simulink model "Just_The_Electrical_model"  (R2016a)
settings: Solver=VariableStepAuto  StartTime=0.0  StopTime=10.0  RelTol=1e-3
values from neighbouring files (symbols this model uses):
  BT = {}    [Electrical_model_settings.m]
  btc = {}    [Electrical_model_settings.m]
  col = {}    [Electrical_model_settings.m]
  elc = {}    [Electrical_model_settings.m]
  ess = {}    [Electrical_model_settings.m]
  fcc = {}    [Electrical_model_settings.m]
  flex = {}    [Electrical_model_settings.m]
  systemBase = {}    [Electrical_model_settings.m]
  wf = {}    [Electrical_model_settings.m]
  wt1 = {}    [Electrical_model_settings.m]
  wt2 = wt1    [Electrical_model_settings.m]
  wt3 = wt1    [Electrical_model_settings.m]
undefined symbols (not defined in the file or in its folder): avr, D1, Delta, DiscIntNeverNeededParam, f2ctrl, governor, interface, Lf1, sm, Ts, Ts_phy, Ts_sim, u0
libraries: powerlib x69, pwrsysBasic x68, simulink_extras x37, pwrsysVICtrl x22, powerlib_meascontrol x19, simulink x8, pwrsysVSrc x5, pwrsysTransf x5, pwrsys-matlab x1
(part 1 of 4)
settings Model: Creator=daniemot  LastModifiedBy=daniemot

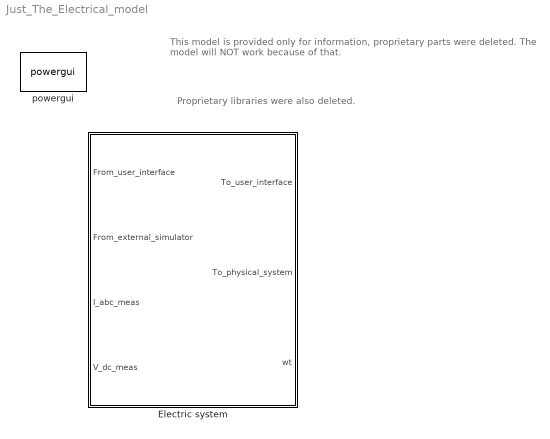
== system Just_The_Electrical_model ==
  note: Proprietary libraries were also deleted.
  note: This model is provided only for information, proprietary parts were deleted.
      | The model will NOT work because of that.
  Electric system : Subsystem
  powergui : powerlib/powergui  Priority=1  SimulationMode=Discrete  SolverType=Tustin  SampleTime=max(Ts_phy,Ts_sim)  frequency=60  SPID=off  DisableSnubberDevices=off  DisableRonSwitches=off  DisableVfSwitches=off  SwTol=0  DisplayEquations=off  Interpol=off  ExternalGateDelay=off  methode=off  Ts=0  FunctionMessages=off  echomessages=off  HookPort=off  EnableUseOfTLC=off  x0status=blocks  frequencyindice=0  Pbase=100e6  ErrMax=1e-4  Iterations=50  UnitsV=kV  UnitsW=MW  buscounter=0  RestoreLinks=warning  ResistiveCurrentMeasurement=off  Frange=[0:2:500]  Ylog=off  Xlog=on  ShowGrid=off  save=off  variable=ZData  structure=0  ZoomFFT=off  StartTime=0.0  cycles=1  DisplayStyle=1  fundamental=60  FreqAxis=off  MaxFrequency=1000  frequencyindicesteady=1  RmsSteady=1  display=off

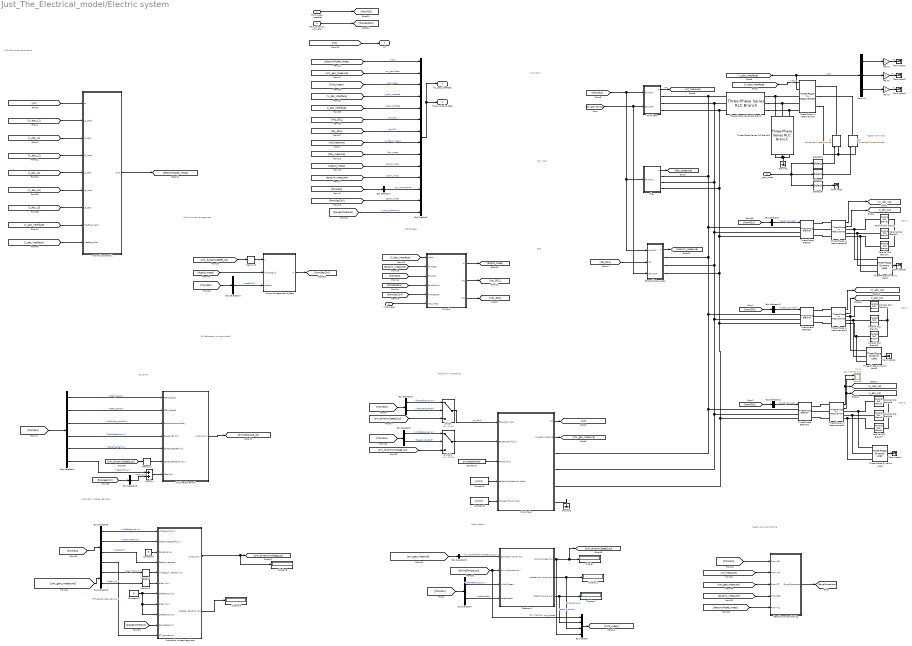
== system Just_The_Electrical_model/Electric system ==
  note: Egston terminals
  note: RMS and power calculation
  note: Automatic voltage regulator
  note: Back emf + reactance
  note: Mech.rotation
  note: Governor
  note: SM Generator (simple model)
  note: Load 3
  note: Load 2
  note: Load 1
  note: Wind
      | farm
  note: Flex
      | load
  note: DC Storage
  note: ESS
  note: Active Power Management
  note: Reactive Power Sharing
  From_user_interface : Inport
  From_external_simulator : Inport  Port=2
  I_abc_meas : Inport  Port=3
  V_dc_meas : Inport  Port=4
  Automatic voltage regulator : Subsystem
  Bus Creator : BusCreator  Inputs=4
  Bus Creator2 : BusCreator  Inputs=14
  Bus Selector1 : BusSelector  OutputSignals=load1_connect
  Bus Selector10 : BusSelector  OutputSignals=sm_backEmfPowerMeasure_pu
  Bus Selector11 : BusSelector  OutputSignals=load2_connect
  Bus Selector12 : BusSelector  OutputSignals=load3_connect
  Bus Selector14 : BusSelector  OutputSignals=resetPMS
  Bus Selector2 : BusSelector  OutputSignals=load1_connect,load2_connect,load3_connect,ESS_connect,WF_connect,WT1_connect,WT2_connect,WT3_connect,Flex_connect,WF_windsim,ESSPHIL_enable,ExtSim_enable,voltRef_ESS_pu,voltRef_WT1_pu,voltRef_WT2_pu,voltRef_WT3_pu,PRef_FC_pu,PRef_ELY_pu,PRef_Batt_pu,PRef_GT_pu  OutputAsBus=on
  Bus Selector3 : BusSelector  OutputSignals=Psec_gt
  Bus Selector4 : BusSelector  OutputSignals=FCRN_Case2,FCRN_Case3,turbDelay_enable,freqReference pu,deltaFreqRef pu,PRef_GT_pu
  Bus Selector5 : BusSelector  OutputSignals=voltReference pu,freezeVoltAtRef
  Bus Selector6 : BusSelector  OutputSignals=freqReference pu,freezeFreqAtRef
  Bus Selector7 : BusSelector  OutputSignals=freqReference pu,resetSpeed
  Bus Selector8 : BusSelector  OutputSignals=voltReference pu,deltaVoltRef pu,resetAVR,GT_ReactiveConsensus
  Bus Selector9 : BusSelector  OutputSignals=Vgen_filt [pu],Qgen_pu
  Constant1 : Constant  Value=sm.phaseInitial  SampleTime=Ts
  Constant12 : Constant  Value=0  SampleTime=Ts
  Constant2 : Constant  Value=[0 0 0]  SampleTime=Ts
  Constant3 : Constant  Value=[0 0 0]  SampleTime=Ts
  Constant4 : Constant  Value=0  SampleTime=Ts
  DC Grid : Subsystem
  Demux1 : Demux  Outputs=3
  Display{,1..3,5} (5 alike) : Display
  ESS_Grid_Converter : Subsystem
  Flex : Subsystem
  Gain1 : Gain
  Gain2 : Gain
  Gain3 : Gain
  Ground1 : powerlib/Elements/Ground  LConnTagsString=a
  Ground3 : powerlib/Elements/Ground  LConnTagsString=a
  IL : powerlib/Electrical Sources/Controlled Current Source  Initialize=on  Source_Type=AC  Amplitude=0  Phase=0  Frequency=0  Measurements=None
  IL1 : powerlib/Electrical Sources/Controlled Current Source  Initialize=on  Source_Type=AC  Amplitude=0  Phase=0  Frequency=0  Measurements=None
  Memory{1..4} (4 alike) : Memory
  Parallel RLC Branch : powerlib/Elements/Parallel RLC Branch  LConnTagsString=a  RConnTagsString=__new0  BranchType=RL  Resistance=load.R(1)/(1-load.ConstPratio(1))  Inductance=load.L(1)/(1-load.ConstPratio(1))  SetiL0=off  InitialCurrent=0  Capacitance=1e-6  Setx0=off  InitialVoltage=0  Measurements=None
  Parallel RLC Branch1 : powerlib/Elements/Parallel RLC Branch  LConnTagsString=a  RConnTagsString=__new0  BranchType=RL  Resistance=load.R(1)/(1-load.ConstPratio(1))  Inductance=load.L(1)/(1-load.ConstPratio(1))  SetiL0=off  InitialCurrent=0  Capacitance=1e-6  Setx0=off  InitialVoltage=0  Measurements=None
  Parallel RLC Branch2 : powerlib/Elements/Parallel RLC Branch  LConnTagsString=a  RConnTagsString=__new0  BranchType=RL  Resistance=load.R(1)/(1-load.ConstPratio(1))  Inductance=load.L(1)/(1-load.ConstPratio(1))  SetiL0=off  InitialCurrent=0  Capacitance=1e-6  Setx0=off  InitialVoltage=0  Measurements=None
  Parallel RLC Branch3 : powerlib/Elements/Parallel RLC Branch  LConnTagsString=a  RConnTagsString=__new0  BranchType=RL  Resistance=load.R(2)/(1-load.ConstPratio(2))  Inductance=load.L(2)/(1-load.ConstPratio(2))  SetiL0=off  InitialCurrent=0  Capacitance=1e-6  Setx0=off  InitialVoltage=0  Measurements=None
  Parallel RLC Branch4 : powerlib/Elements/Parallel RLC Branch  LConnTagsString=a  RConnTagsString=__new0  BranchType=RL  Resistance=load.R(2)/(1-load.ConstPratio(2))  Inductance=load.L(2)/(1-load.ConstPratio(2))  SetiL0=off  InitialCurrent=0  Capacitance=1e-6  Setx0=off  InitialVoltage=0  Measurements=None
  Parallel RLC Branch5 : powerlib/Elements/Parallel RLC Branch  LConnTagsString=a  RConnTagsString=__new0  BranchType=RL  Resistance=load.R(2)/(1-load.ConstPratio(2))  Inductance=load.L(2)/(1-load.ConstPratio(2))  SetiL0=off  InitialCurrent=0  Capacitance=1e-6  Setx0=off  InitialVoltage=0  Measurements=None
  Parallel RLC Branch6 : powerlib/Elements/Parallel RLC Branch  LConnTagsString=a  RConnTagsString=__new0  BranchType=RL  Resistance=load.R(3)/(1-load.ConstPratio(3))  Inductance=load.L(3)/(1-load.ConstPratio(3))  SetiL0=off  InitialCurrent=0  Capacitance=1e-6  Setx0=off  InitialVoltage=0  Measurements=None
  Parallel RLC Branch7 : powerlib/Elements/Parallel RLC Branch  LConnTagsString=a  RConnTagsString=__new0  BranchType=RL  Resistance=load.R(3)/(1-load.ConstPratio(3))  Inductance=load.L(3)/(1-load.ConstPratio(3))  SetiL0=off  InitialCurrent=0  Capacitance=1e-6  Setx0=off  InitialVoltage=0  Measurements=None
  Parallel RLC Branch8 : powerlib/Elements/Parallel RLC Branch  LConnTagsString=a  RConnTagsString=__new0  BranchType=RL  Resistance=load.R(3)/(1-load.ConstPratio(3))  Inductance=load.L(3)/(1-load.ConstPratio(3))  SetiL0=off  InitialCurrent=0  Capacitance=1e-6  Setx0=off  InitialVoltage=0  Measurements=None
  Power Management System : Subsystem
  Reactive power sharing : Subsystem
  Rotation1 : Subsystem
  SM_simple : Subsystem
  Scope : Scope  Commented=on  NumInputPorts=2
  Selector6 : Selector  InputPortWidth=3  IndexOptions=Index vector (dialog)  Indices=[1]  OutputSizes=1
  Selector7 : Selector  InputPortWidth=3  IndexOptions=Index vector (dialog)  Indices=2  OutputSizes=1
  Selector8 : Selector  InputPortWidth=3  IndexOptions=Index vector (dialog)  Indices=3  OutputSizes=1
  Switch : Switch  Threshold=0.5
  Switch1 : Switch  Threshold=0.5
  Terminator{,1..6} (7 alike) : Terminator
  Three-Phase Dynamic Load : powerlib/Elements/Three-Phase Dynamic Load  NominalVoltage=[ systemBase.Vn systemBase.fn ]  ActiveReactivePowers=[load.P(3)*load.ConstPratio(3) load.P(3)*tan(acos(load.cosphi(3)))*load.ConstPratio(3)]  PositiveSequence=[1 0]  ExternalControl=off  NpNq=[0 2]  TimeConstants="[0  0  0  0]"  MinimumVoltage=0.7  LoadFlowParameters=[4,0,0,0,0]
  Three-Phase Dynamic Load1 : powerlib/Elements/Three-Phase Dynamic Load  NominalVoltage=[ systemBase.Vn systemBase.fn ]  ActiveReactivePowers=[load.P(1)*load.ConstPratio(1) load.P(1)*tan(acos(load.cosphi(3)))*load.ConstPratio(1)]  PositiveSequence=[1 0]  ExternalControl=off  NpNq=[0 2]  TimeConstants="[0  0  0  0]"  MinimumVoltage=0.7  LoadFlowParameters=[4,0,0,0,0]
  Three-Phase Dynamic Load2 : powerlib/Elements/Three-Phase Dynamic Load  NominalVoltage=[ systemBase.Vn systemBase.fn ]  ActiveReactivePowers=[load.P(2)*load.ConstPratio(2) load.P(2)*tan(acos(load.cosphi(2)))*load.ConstPratio(2)]  PositiveSequence=[1 0]  ExternalControl=off  NpNq=[0 2]  TimeConstants="[0  0  0  0]"  MinimumVoltage=0.7  LoadFlowParameters=[4,0,0,0,0]
  Three-Phase Series RLC Branch : powerlib/Elements/Three-Phase Series RLC Branch  LConnTagsString=A|B|C  RConnTagsString=A|B|C  BranchType=R  Resistance=interface.Rs  Inductance=1e-3  Capacitance=1e-6  Measurements=None
  Three-Phase Series RLC Branch1 : powerlib/Elements/Three-Phase Series RLC Branch  LConnTagsString=A|B|C  RConnTagsString=A|B|C  BranchType=R  Resistance=interface.Rp  Inductance=1e-3  Capacitance=1e-6  Measurements=None
  Three-Phase V-I Measurement{,1..3} (4 alike) : powerlib/Measurements/Three-Phase V-I Measurement  VoltageMeasurement=phase-to-ground  SetLabelV=off  LabelV=Vabc  Vpu=off  VpuLL=off  CurrentMeasurement=yes  SetLabelI=off  LabelI=Iabc  Ipu=off  Pbase=100e6  Vbase=500e3  OutputType=Complex  PhasorSimulation=off  PSBequivalent=0
  Three-Phase Breaker : powerlib/Elements/Three-Phase Breaker  InitialState=open  SwitchA=on  SwitchB=on  SwitchC=on  SwitchTimes="[4/60  10/60]"  External=on  BreakerResistance=0.001  SnubberResistance=1e6  SnubberCapacitance=inf  Measurements=None
  Three-Phase Breaker1 : powerlib/Elements/Three-Phase Breaker  InitialState=open  SwitchA=on  SwitchB=on  SwitchC=on  SwitchTimes="[4/60  10/60]"  External=on  BreakerResistance=0.001  SnubberResistance=1e6  SnubberCapacitance=inf  Measurements=None
  Three-Phase Breaker2 : powerlib/Elements/Three-Phase Breaker  InitialState=open  SwitchA=on  SwitchB=on  SwitchC=on  SwitchTimes="[4/60  10/60]"  External=on  BreakerResistance=0.001  SnubberResistance=1e6  SnubberCapacitance=inf  Measurements=None
  Turbine Governor1 : Subsystem
  Wind Farm : Subsystem
  pRef_pu : Sum
  rms and power calc : Subsystem
  To_user_interface : Outport
  To_physical_system : Outport  Port=2
  wt : Outport  Port=3
  wires:
  Bus Selector12/1 -> Three-Phase Breaker2/1  "<load3_connect>"
  [fromGUI] -> Bus Selector12/1
  Bus Selector11/1 -> Three-Phase Breaker1/1  "<load2_connect>"
  [fromGUI] -> Bus Selector11/1
  Bus Selector1/1 -> Three-Phase Breaker/1  "<load1_connect>"
  [fromGUI] -> Bus Selector1/1
  Three-Phase V-I Measurement2/1 -> Scope/1, [V_abc_L3]
  Three-Phase V-I Measurement2/2 -> Scope/2, [I_abc_L3]
  Three-Phase V-I Measurement1/1 -> [V_abc_L2]
  Three-Phase V-I Measurement1/2 -> [I_abc_L2]
  Three-Phase V-I Measurement3/2 -> [I_abc_L1]
  Three-Phase V-I Measurement3/1 -> [V_abc_L1]
  Bus Selector10/1 -> Rotation1/1(generator power (pu))  "<sm_backEmfPowerMeasure_pu>"
  [sm_gen_measure] -> Bus Selector10/1
  Bus Selector9/1 -> Memory2/1  "<Vgen_filt [pu]>"
  SM_simple/1(wt1) -> [wt]
  Memory2/1 -> Automatic voltage regulator/5(voltage_feedback (pu))
  Bus Selector4/3 -> Turbine Governor1/3(EnableActuatorDelay)  "<turbDelay_enable>"
  Bus Selector7/2 -> Rotation1/4(resetSpeed)  "<resetSpeed>"
  Bus Selector5/2 -> Switch1/2  "<freezeVoltAtRef>"
  Bus Selector6/2 -> Switch/2  "<freezeFreqAtRef>"
  Constant12/1 -> Automatic voltage regulator/9(pRefDroop (pu)), Automatic voltage regulator/8(pGen (pu)), Automatic voltage regulator/7(qRefDroop (pu))
  Constant4/1 -> Automatic voltage regulator/3(Reset_value)
  Bus Selector8/3 -> Automatic voltage regulator/4(Reset_integrator)  "<resetAVR>"
  Bus Selector8/2 -> Automatic voltage regulator/2(deltaVoltageRef (pu))  "<deltaVoltRef pu>"
  Bus Selector4/5 -> Turbine Governor1/5(deltaSpeedRef (pu))  "<deltaFreqRef pu>"
  Bus Selector4/4 -> Turbine Governor1/4(Speed_ref (pu))  "<freqReference pu>"
  Bus Selector8/1 -> Automatic voltage regulator/1(Voltage_ref (pu))  "<voltReference pu>"
  [fromGUI] -> Bus Selector8/1
  Bus Selector7/1 -> Rotation1/3(InitialSpeed)  "<freqReference pu>"
  [fromGUI] -> Bus Selector7/1
  Bus Selector6/1 -> Switch/1  "<freqReference pu>"
  [fromGUI] -> Bus Selector6/1
  Bus Selector5/1 -> Switch1/1  "<voltReference pu>"
  [fromGUI] -> Bus Selector5/1
  [fromGUI] -> Bus Selector4/1
  [drivingTorque_pu] -> Bus Creator/1, Rotation1/2(driving torque (pu))  "driving_torque"
  Turbine Governor1/1(output (pu)) -> [drivingTorque_pu]
  [sm_gen_measure] -> Bus Selector9/1
  Automatic voltage regulator/2(voltageRefActual (pu)) -> Display5/1
  Automatic voltage regulator/1(output (pu)) -> Display3/1, [sm_dynamicVoltage_pu]
  Memory1/1 -> Turbine Governor1/6(Speed_feedback (pu))
  [sm_dynamicSpeed_pu] -> Memory1/1
  [sm_dynamicVoltage_pu] -> Switch1/3
  [sm_dynamicSpeed_pu] -> Switch/3
  Rotation1/3(electric torque (pu)) -> Bus Creator/2, Display2/1  "electric_torque"
  Rotation1/2(mechanical torque (pu)) -> Bus Creator/3, Display1/1  "accel_torque"
  Rotation1/1(turbine speed (pu)) -> Bus Creator/4, Display/1, [sm_dynamicSpeed_pu]  "turb_speed"
  Switch1/1 -> SM_simple/2(GenBackEmf [pu])
  Bus Creator2/1 -> To_user_interface/1, To_physical_system/1
  SM_simple/2(sm_gen_measure) -> [sm_gen_measure]
  Constant3/1 -> SM_simple/5(phaseSkiftIndividual)
  Constant2/1 -> SM_simple/4(deltaAmplitudeIndividual)
  Constant1/1 -> SM_simple/3(Phase [rad])
  Switch/1 -> SM_simple/1(Frequency [pu])  "sm_freq"
  From_user_interface/1 -> [fromGUI]
  Gain3/1 -> Terminator3/1  "Ic"
  Demux1/3 -> Gain3/1
  Gain2/1 -> Terminator2/1  "Ib"
  Demux1/2 -> Gain2/1
  Gain1/1 -> Terminator1/1  "Ia"
  Demux1/1 -> Gain1/1
  Selector7/1 -> IL1/1
  Three-Phase V-I Measurement/2 -> Demux1/1, [I_abc_interface]  "I_abc"
  Selector8/1 -> Terminator/1
  I_abc_meas/1 -> Selector6/1, Selector7/1, Selector8/1
  Three-Phase V-I Measurement/1 -> [V_abc_interface]  "V_abc"
  Selector6/1 -> IL/1
  [wt] -> wt/1
  [wt] -> rms and power calc/1(wt)
  [V_abc_L1] -> rms and power calc/2(L1_Vabc)
  [I_abc_L1] -> rms and power calc/3(L1_Iabc)
  [V_abc_L2] -> rms and power calc/4(L2_Vabc)
  [I_abc_L2] -> rms and power calc/5(L2_Iabc)
  [V_abc_L3] -> rms and power calc/6(L3_Vabc)
  [I_abc_L3] -> rms and power calc/7(L3_Iabc)
  [V_abc_interface] -> rms and power calc/8(Interface_Vabc)
  [I_abc_interface] -> rms and power calc/9(Interface_Iabc)
  rms and power calc/1(Out1) -> [electricModel_meas]
  [electricModel_meas] -> Bus Creator2/1  "loads"
  [sm_gen_measure] -> Bus Creator2/2  "sm_gemMeas"
  Wind Farm/1(m) -> [wf_measure]  "WF"
  [fromGUI] -> ESS_Grid_Converter/1(fromGUI), Flex/1(fromGUI), Wind Farm/1(fromGUI)
  Flex/1(m) -> [flex_measure]
  [V_abc_interface] -> Bus Creator2/4  "V_abc_interface"
  [I_abc_interface] -> Bus Creator2/5  "I_abc_interface"
  [Idc_DCL] -> Bus Creator2/7  "Idc_DCL"
  [Vdc_DCL] -> Bus Creator2/6  "Vdc_DCL"
  [wf_measure] -> Bus Creator2/8  "windfarm_meas"
  [flex_measure] -> Bus Creator2/9  "flex_meas"
  V_dc_meas/1 -> DC Grid/6(Vdc_meas)
  [dcgrid_meas] -> Bus Creator2/10  "dcgrid_meas"
  [fromGUI] -> DC Grid/3(fromGUI)
  DC Grid/1(m) -> [dcgrid_meas]
  DC Grid/2(Idc) -> [Idc_DCL]
  DC Grid/3(Vdc) -> [Vdc_DCL]
  From_external_simulator/1 -> [fromExtSim]
  [fromExtSim] -> DC Grid/4(fromExtSim)
  ESS_Grid_Converter/1(m) -> [esssim_measure]
  [esssim_measure] -> Bus Creator2/11  "essim_meas"
  [esssim_measure] -> DC Grid/2(fromESS)
  [fromSecCtrl] -> DC Grid/5(fromSecCtrl)
  [fromSecCtrl] -> Bus Selector3/1
  [sm_dynamicSpeed_pu] -> Memory3/1
  Power Management System/1(m) -> [fromSecCtrl]
  Memory3/1 -> Power Management System/1(w)
  [fromGUI] -> Bus Selector2/1
  Bus Selector2/1 -> Bus Creator2/12  "gui_commands"
  [fromSecCtrl] -> Bus Creator2/13  "secCtrl_meas"
  [dcgrid_meas] -> Power Management System/2(fromDCgrid)
  Bus Selector3/1 -> pRef_pu/2  "<Psec_gt>"
  Bus Selector4/6 -> pRef_pu/1  "<PRef_GT_pu>"
  pRef_pu/1 -> Turbine Governor1/7(pRef (pu))
  [Idc_DCL] -> ESS_Grid_Converter/2(Idc)
  [fromGUI] -> Bus Selector14/1
  Bus Selector14/1 -> Power Management System/3(resetInt)  "<resetPMS>"
  Three-Phase Dynamic Load/1 -> Terminator4/1
  Three-Phase Dynamic Load1/1 -> Terminator5/1
  [V_abc_interface] -> DC Grid/1(Vabc)
  [fromGUI] -> Reactive power sharing/1(From GUI)
  Reactive power sharing/1(QavgConsensus) -> [QavgConsensus]
  [wf_measure] -> Reactive power sharing/2(From WF)
  [QavgConsensus] -> ESS_Grid_Converter/3(QavgWF), Wind Farm/2(QavgWF)
  [sm_gen_measure] -> Reactive power sharing/3(From GT)
  [esssim_measure] -> Reactive power sharing/4(From ESS)
  [electricModel_meas] -> Reactive power sharing/5(From HIL)
  Bus Selector9/2 -> Memory4/1  "<Qgen_pu>"
  Memory4/1 -> Automatic voltage regulator/6(qGen (pu))
  [QavgConsensus] -> Automatic voltage regulator/10(QavgSetpoint)
  Bus Selector8/4 -> Automatic voltage regulator/11(GT_consensus)  "<GT_ReactiveConsensus>"
  [QavgConsensus] -> Bus Creator2/14  "q_avg_consensus"
  Bus Selector4/2 -> Turbine Governor1/2(FCRN_Case3)  "<FCRN_Case3>"
  Bus Selector4/1 -> Turbine Governor1/1(FCRN_Case2)  "<FCRN_Case2>"
  Three-Phase Dynamic Load2/1 -> Terminator6/1
  Bus Creator/1 -> [turb_meas]
  [turb_meas] -> Bus Creator2/3  "turb_meas"
  connections:
  Ground3/LConn1 -- SM_simple/RConn4
  Three-Phase V-I Measurement2/LConn3 -- Three-Phase Breaker2/RConn3
  Three-Phase V-I Measurement2/LConn2 -- Three-Phase Breaker2/RConn2
  Three-Phase V-I Measurement2/LConn1 -- Three-Phase Breaker2/RConn1
  Three-Phase V-I Measurement1/LConn1 -- Three-Phase Breaker1/RConn1
  Three-Phase V-I Measurement1/LConn2 -- Three-Phase Breaker1/RConn2
  Three-Phase V-I Measurement1/LConn3 -- Three-Phase Breaker1/RConn3
  Three-Phase V-I Measurement3/LConn3 -- Three-Phase Breaker/RConn3
  Three-Phase V-I Measurement3/LConn2 -- Three-Phase Breaker/RConn2
  Three-Phase V-I Measurement3/LConn1 -- Three-Phase Breaker/RConn1
  Parallel RLC Branch1/LConn1 -- Three-Phase Dynamic Load1/LConn3 -- Three-Phase V-I Measurement3/RConn3
  Three-Phase V-I Measurement3/RConn2 -- Three-Phase Dynamic Load1/LConn2 -- Parallel RLC Branch2/LConn1
  Parallel RLC Branch/LConn1 -- Three-Phase Dynamic Load1/LConn1 -- Three-Phase V-I Measurement3/RConn1
  Parallel RLC Branch/RConn1 -- Parallel RLC Branch1/RConn1 -- Parallel RLC Branch2/RConn1
  Three-Phase Breaker/LConn3 -- ESS_Grid_Converter/RConn3 -- Three-Phase Breaker2/LConn3 -- SM_simple/RConn3 -- Three-Phase Breaker1/LConn3 -- Flex/RConn3 -- Wind Farm/RConn3 -- Three-Phase Series RLC Branch/LConn3
  Three-Phase Breaker2/LConn2 -- SM_simple/RConn2 -- Three-Phase Breaker1/LConn2 -- ESS_Grid_Converter/RConn2 -- Three-Phase Breaker/LConn2 -- Flex/RConn2 -- Wind Farm/RConn2 -- Three-Phase Series RLC Branch/LConn2
  Three-Phase Breaker/LConn1 -- Three-Phase Breaker2/LConn1 -- SM_simple/RConn1 -- Three-Phase Breaker1/LConn1 -- ESS_Grid_Converter/RConn1 -- Flex/RConn1 -- Wind Farm/RConn1 -- Three-Phase Series RLC Branch/LConn1
  Three-Phase Series RLC Branch/RConn1 -- Three-Phase V-I Measurement/RConn1 -- Three-Phase Series RLC Branch1/RConn1
  Three-Phase Series RLC Branch/RConn2 -- Three-Phase V-I Measurement/RConn2 -- Three-Phase Series RLC Branch1/RConn2
  Three-Phase Series RLC Branch/RConn3 -- Three-Phase V-I Measurement/RConn3 -- Three-Phase Series RLC Branch1/RConn3
  Three-Phase Series RLC Branch1/LConn2 -- Three-Phase Series RLC Branch1/LConn3 -- Ground1/LConn1 -- Three-Phase Series RLC Branch1/LConn1
  IL/LConn1 -- IL1/LConn1 -- Three-Phase V-I Measurement/LConn3
  Parallel RLC Branch3/RConn1 -- Parallel RLC Branch5/RConn1 -- Parallel RLC Branch4/RConn1
  Three-Phase V-I Measurement1/RConn1 -- Three-Phase Dynamic Load2/LConn1 -- Parallel RLC Branch3/LConn1
  Three-Phase V-I Measurement1/RConn2 -- Parallel RLC Branch4/LConn1 -- Three-Phase Dynamic Load2/LConn2
  Three-Phase V-I Measurement1/RConn3 -- Parallel RLC Branch5/LConn1 -- Three-Phase Dynamic Load2/LConn3
  Parallel RLC Branch8/RConn1 -- Parallel RLC Branch7/RConn1 -- Parallel RLC Branch6/RConn1
  Three-Phase Dynamic Load/LConn1 -- Three-Phase V-I Measurement2/RConn1 -- Parallel RLC Branch6/LConn1
  Three-Phase Dynamic Load/LConn2 -- Parallel RLC Branch8/LConn1 -- Three-Phase V-I Measurement2/RConn2
  Three-Phase Dynamic Load/LConn3 -- Parallel RLC Branch7/LConn1 -- Three-Phase V-I Measurement2/RConn3
  Three-Phase V-I Measurement/LConn2 -- IL1/RConn1
  Three-Phase V-I Measurement/LConn1 -- IL/RConn1

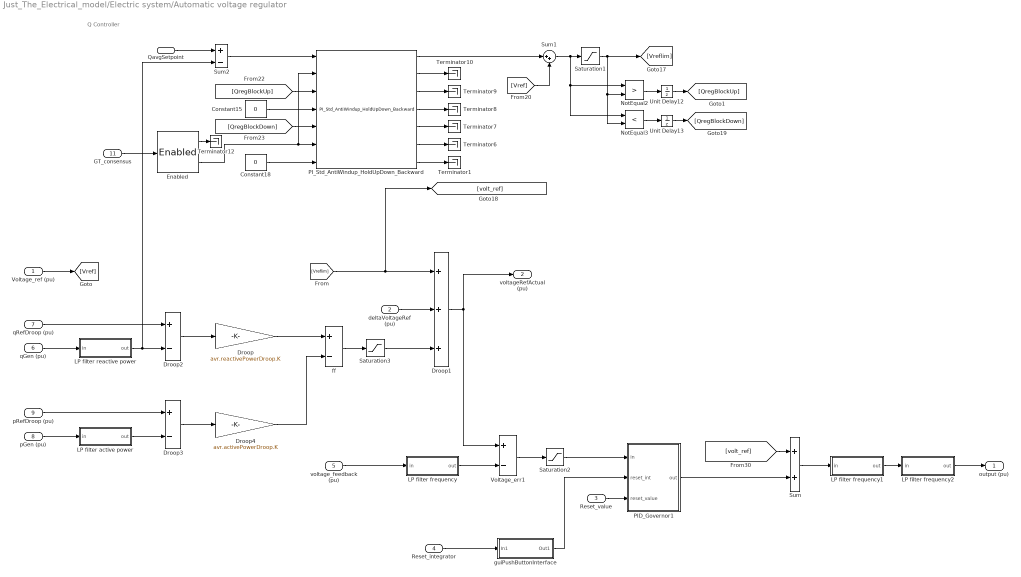
== system Just_The_Electrical_model/Electric system/Automatic voltage regulator ==
  note: Q Controller
  Voltage_ref (pu) : Inport
  deltaVoltageRef (pu) : Inport  Port=2
  Reset_value : Inport  Port=3
  Reset_integrator : Inport  Port=4
  voltage_feedback (pu) : Inport  Port=5
  qGen (pu) : Inport  Port=6
  qRefDroop (pu) : Inport  Port=7
  pGen (pu) : Inport  Port=8
  pRefDroop (pu) : Inport  Port=9
  QavgSetpoint : Inport  Port=10
  GT_consensus : Inport  Port=11
  Constant15 : Constant  Value=0
  Constant18 : Constant  Value=0
  Droop : Gain  Gain=avr.reactivePowerDroop.K
  Droop1 : Sum  Inputs=+++
  Droop2 : Sum  Inputs=+-
  Droop3 : Sum  Inputs=+-
  Droop4 : Gain  Gain=avr.activePowerDroop.K
  Enabled : pwrsysBasic/Enabled
  LP filter active power : Subsystem  mask(Discrete first order low pass filter){tau=avr.LPfilterPowerMeasurementDroop.T, Ts=Ts, x0=0, y0=0}
      mask prompts: tau "Filter time constant [s]"; Ts "Sampling time [s]"; x0 "Initial input"; y0 "Initial output"
      mask help: Discrete first order low pass filter derived from a continous filter by bilinear transformation.
  LP filter frequency : Subsystem  mask(Discrete first order low pass filter){tau=avr.LPfilterVoltageMeasurement.T, Ts=Ts, x0=0, y0=0}
      mask prompts: tau "Filter time constant [s]"; Ts "Sampling time [s]"; x0 "Initial input"; y0 "Initial output"
      mask help: Discrete first order low pass filter derived from a continous filter by bilinear transformation.
  LP filter frequency1 : Subsystem  mask(Discrete first order low pass filter){tau=avr.fieldWinding.T1, Ts=Ts, x0=avr.init, y0=avr.init}
      mask prompts: tau "Filter time constant [s]"; Ts "Sampling time [s]"; x0 "Initial input"; y0 "Initial output"
      mask help: Discrete first order low pass filter derived from a continous filter by bilinear transformation.
  LP filter frequency2 : Subsystem  mask(Discrete first order low pass filter){tau=avr.fieldWinding.T2, Ts=Ts, x0=avr.init, y0=avr.init}
      mask prompts: tau "Filter time constant [s]"; Ts "Sampling time [s]"; x0 "Initial input"; y0 "Initial output"
      mask help: Discrete first order low pass filter derived from a continous filter by bilinear transformation.
  LP filter reactive power : Subsystem  mask(Discrete first order low pass filter){tau=avr.LPfilterReactivePowerMeasurementDroop.T, Ts=Ts, x0=0, y0=0}
      mask prompts: tau "Filter time constant [s]"; Ts "Sampling time [s]"; x0 "Initial input"; y0 "Initial output"
      mask help: Discrete first order low pass filter derived from a continous filter by bilinear transformation.
  NotEqual2 : RelationalOperator  Operator=>  OutDataTypeStr=boolean
  NotEqual3 : RelationalOperator  Operator=<  OutDataTypeStr=boolean
  PID_Governor1 : Subsystem  mask(Discrete PI with parallel form){kp=avr.kP, ki=avr.kI, kd=avr.kd, Tlp=avr.derivativeLP, xi=0, up_sat_limit=avr.saturationUpper, low_sat_limit=avr.saturationLower}
      mask prompts: kp "Proportional gain"; ki "Integral gain"; kd "Derivative gain"; Tlp "Derivative LP filter T"; xi "Initial condition integrator"; up_sat_limit "Saturation upper limit"; low_sat_limit "Saturation lower limit"
      mask help: Discrete PI in parallel form with saturation on the integrator and on the output. The upper and the lower saturation limits are fixed.
  PI_Std_AntiWindup_HoldUpDown_Backward : pwrsysBasic/PI_Std_AntiWindup_HoldUpDown_Backward  Ts=avr.Qctrl.Ts_control  Kg=avr.Qctrl.Kg  Kp=avr.Qctrl.Kp  Ti=avr.Qctrl.Ti  outMax=avr.Qctrl.deltaUmaxPos  outMin=avr.Qctrl.deltaUmaxNeg
  Saturation1 : Saturate  UpperLimit=avr.Qctrl.Umax  LowerLimit=avr.Qctrl.Umin
  Saturation2 : Saturate  UpperLimit=avr.ErrMax  LowerLimit=avr.ErrMin
  Saturation3 : Saturate  UpperLimit=avr.droopSaturationUpper  LowerLimit=avr.droopSaturationLower
  Sum : Sum
  Sum1 : Sum  Inputs=|++
  Sum2 : Sum  Inputs=+-
  Terminator{1,6..10,12} (7 alike) : Terminator
  Unit Delay12 : UnitDelay  SampleTime=avr.Qctrl.Ts_control
  Unit Delay13 : UnitDelay  SampleTime=avr.Qctrl.Ts_control
  Voltage_err1 : Sum  Inputs=+-
  ff : Sum  Inputs=+-
  guiPushButtonInterface : Subsystem
  output (pu) : Outport
  voltageRefActual (pu) : Outport  Port=2
  wires:
  guiPushButtonInterface/1(Out1) -> PID_Governor1/2(reset_int)
  Reset_value/1 -> PID_Governor1/3(reset_value)
  Sum/1 -> LP filter frequency1/1(in)
  [volt_ref] -> Sum/1
  ff/1 -> Saturation3/1
  Droop4/1 -> ff/2
  Droop3/1 -> Droop4/1
  LP filter active power/1(out) -> Droop3/2
  pRefDroop (pu)/1 -> Droop3/1
  pGen (pu)/1 -> LP filter active power/1(in)
  LP filter frequency1/1(out) -> LP filter frequency2/1(in)
  Saturation3/1 -> Droop1/3
  Saturation2/1 -> PID_Governor1/1(in)
  deltaVoltageRef (pu)/1 -> Droop1/2
  Droop2/1 -> Droop/1
  qRefDroop (pu)/1 -> Droop2/1
  qGen (pu)/1 -> LP filter reactive power/1(in)
  Voltage_err1/1 -> Saturation2/1
  Droop/1 -> ff/1
  LP filter frequency/1(out) -> Voltage_err1/2
  PID_Governor1/1(out) -> Sum/2
  Reset_integrator/1 -> guiPushButtonInterface/1(In1)
  Droop1/1 -> voltageRefActual (pu)/1, Voltage_err1/1
  voltage_feedback (pu)/1 -> LP filter frequency/1(in)
  [Vreflim] -> Droop1/1, [volt_ref]
  [Vref] -> Sum1/2
  Sum1/1 -> NotEqual3/1, NotEqual2/1, Saturation1/1
  Saturation1/1 -> NotEqual3/2, NotEqual2/2, [Vreflim]
  QavgSetpoint/1 -> Sum2/1
  LP filter reactive power/1(out) -> Sum2/2, Droop2/2
  GT_consensus/1 -> Enabled/1
  Sum2/1 -> PI_Std_AntiWindup_HoldUpDown_Backward/1
  [QregBlockUp] -> PI_Std_AntiWindup_HoldUpDown_Backward/3
  Constant15/1 -> PI_Std_AntiWindup_HoldUpDown_Backward/4
  [QregBlockDown] -> PI_Std_AntiWindup_HoldUpDown_Backward/5
  Enabled/2 -> PI_Std_AntiWindup_HoldUpDown_Backward/2, PI_Std_AntiWindup_HoldUpDown_Backward/6
  Constant18/1 -> PI_Std_AntiWindup_HoldUpDown_Backward/7
  PI_Std_AntiWindup_HoldUpDown_Backward/7 -> Terminator1/1
  PI_Std_AntiWindup_HoldUpDown_Backward/6 -> Terminator6/1
  PI_Std_AntiWindup_HoldUpDown_Backward/5 -> Terminator7/1
  PI_Std_AntiWindup_HoldUpDown_Backward/4 -> Terminator8/1
  PI_Std_AntiWindup_HoldUpDown_Backward/3 -> Terminator9/1
  PI_Std_AntiWindup_HoldUpDown_Backward/2 -> Terminator10/1
  NotEqual2/1 -> Unit Delay12/1
  Unit Delay12/1 -> [QregBlockUp]
  NotEqual3/1 -> Unit Delay13/1
  Unit Delay13/1 -> [QregBlockDown]
  PI_Std_AntiWindup_HoldUpDown_Backward/1 -> Sum1/1
  Enabled/1 -> Terminator12/1
  Voltage_ref (pu)/1 -> [Vref]
  LP filter frequency2/1(out) -> output (pu)/1

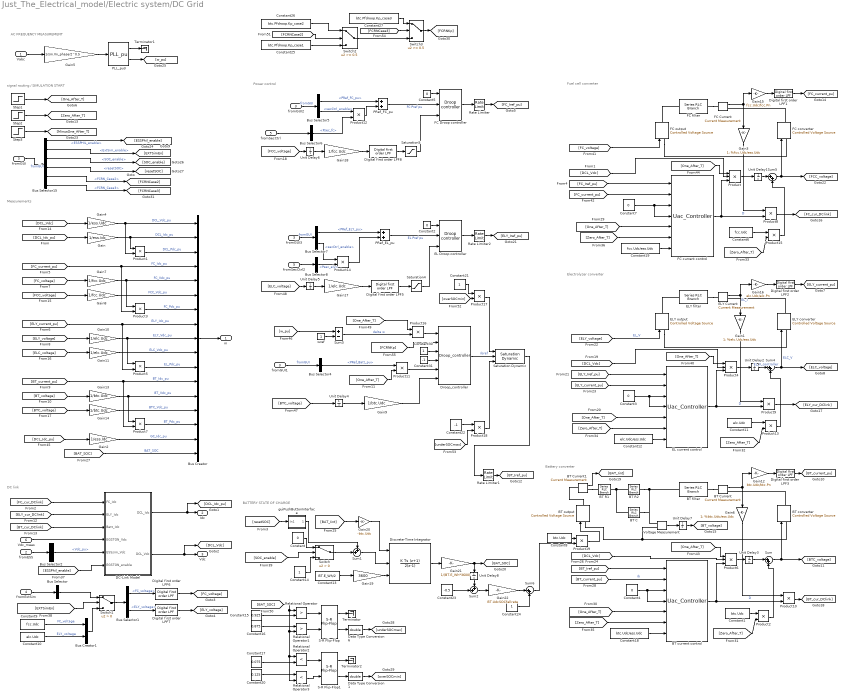
== system Just_The_Electrical_model/Electric system/DC Grid ==
  note: BATTERY STATE OF CHARGE
  note: signal routing / SIMULATION START
  note: AC FREQUENCY MEASUREMENT
  note: Power control
  note: Measurements
  note: DC link
  note: Fuel cell converter
  note: Electrolyzer converter
  note: Battery converter
  Vabc : Inport
  fromESS : Inport  Port=2
  fromGUI : Inport  Port=3
  fromExtSim : Inport  Port=4
  fromSecCtrl : Inport  Port=5
  Vdc_meas : Inport  Port=6
  BT C : powerlib/Elements/Series RLC Branch  LConnTagsString=__new0  RConnTagsString=__new0  BranchType=C  Resistance=BT.C  Inductance=btc.filter.L  SetiL0=on  InitialCurrent=0  Capacitance=BT.C  Setx0=off  InitialVoltage=0  Measurements=None
  BT Current : powerlib/Measurements/Current Measurement  PhasorSimulation=off  OutputType=Complex  PSBequivalent=0
  BT Current1 : powerlib/Measurements/Current Measurement  PhasorSimulation=off  OutputType=Complex  PSBequivalent=0
  BT R1 : powerlib/Elements/Series RLC Branch  LConnTagsString=__new0  RConnTagsString=__new0  BranchType=R  Resistance=BT.R1  Inductance=btc.filter.L  SetiL0=on  InitialCurrent=0  Capacitance=1e-6  Setx0=off  InitialVoltage=0  Measurements=None
  BT R2 : powerlib/Elements/Series RLC Branch  LConnTagsString=__new0  RConnTagsString=__new0  BranchType=R  Resistance=BT.R2  Inductance=btc.filter.L  SetiL0=on  InitialCurrent=0  Capacitance=1e-6  Setx0=off  InitialVoltage=0  Measurements=None
  BT converter : powerlib/Electrical Sources/Controlled Voltage Source  Initialize=on  Source_Type=DC  Amplitude=fcc.Udc  Phase=0  Frequency=0  Measurements=None
  BT current control : pwrsysVICtrl/Uac_Controller  Ts=Ts  Kg=btc.CurrCont.Kg  Kp=btc.CurrCont.Kp  Ti=btc.CurrCont.Ti  PI_max=btc.CurrCont.PImax  PI_min=btc.CurrCont.PImin
  BT filter : powerlib/Elements/Series RLC Branch  LConnTagsString=__new0  RConnTagsString=__new0  BranchType=RL  Resistance=btc.filter.R  Inductance=btc.filter.L  SetiL0=on  InitialCurrent=0  Capacitance=1e-6  Setx0=off  InitialVoltage=0  Measurements=None
  BT output : powerlib/Electrical Sources/Controlled Voltage Source  Initialize=on  Source_Type=DC  Amplitude=fcc.Udc  Phase=0  Frequency=0  Measurements=None
  Bus Creator : BusCreator  Inputs=17
  Bus Creator1 : BusCreator  Inputs=2
  Bus Selector : BusSelector  OutputSignals=FC_voltage,ELY_voltage  OutputAsBus=on
  Bus Selector1 : BusSelector  OutputSignals=FC_voltage,ELY_voltage
  Bus Selector15 : BusSelector  OutputSignals=ESSPHIL_enable,ExtSim_enable,SOC_enable,resetSOC,FCRN_Case2,FCRN_Case3
  Bus Selector2 : BusSelector  OutputSignals=Vdc_pu
  Bus Selector4 : BusSelector  OutputSignals=PRef_Batt_pu
  Bus Selector5 : BusSelector  OutputSignals=PRef_FC_pu,secCtrl_enable
  Bus Selector6 : BusSelector  OutputSignals=Psec_fc
  Bus Selector7 : BusSelector  OutputSignals=PRef_ELY_pu,secCtrl_enable
  Bus Selector8 : BusSelector  OutputSignals=Psec_ely
  Constant : Constant  Value=0
  Constant1 : Constant  Value=btc.Udc  SampleTime=Ts
  Constant10 : Constant  Value=elc.Udc  SampleTime=Ts
  Constant11 : Constant  Value=elc.Udc  SampleTime=Ts
  Constant12 : Constant  Value=elc.Udc/ess.Udc  SampleTime=Ts
  Constant13 : Constant  Value=BT.E_Wh/2  SampleTime=Ts
  Constant14 : Constant
  Constant15 : Constant  Value=0.925
  Constant16 : Constant  Value=0.875
  Constant17 : Constant  Value=0.075
  Constant18 : Constant  Value=btc.Udc/ess.Udc  SampleTime=Ts
  Constant19 : Constant  Value=fcc.Udc/ess.Udc  SampleTime=Ts
  Constant{2..5,7} (5 alike) : Constant  Value=0  SampleTime=Ts
  Constant20 : Constant  Value=0.125
  Constant21 : Constant
  Constant22 : Constant  Value=-1
  Constant23 : Constant  Value=-0.5
  Constant24 : Constant
  Constant25 : Constant  Value=btc.Pfdroop.Kp_case1  SampleTime=-1
  Constant26 : Constant  Value=btc.Pfdroop.Kp_case2  SampleTime=-1
  Constant27 : Constant  Value=btc.Pfdroop.Kp_case3  SampleTime=-1
  Constant30 : Constant  SampleTime=Ts
  Constant31 : Constant  Value=-1  SampleTime=Ts
  Constant6 : Constant  Value=fcc.Udc  SampleTime=Ts
  Constant8 : Constant  Value=btc.Udc  SampleTime=Ts
  Constant9 : Constant  Value=fcc.Udc  SampleTime=Ts
  DC-Link Model : Subsystem
  Data Type Conversion1 : DataTypeConversion  OutDataTypeStr=double  RndMeth=Round
  Data Type Conversion6 : DataTypeConversion  OutDataTypeStr=double  RndMeth=Round
  Digital first order LPF1 : pwrsysBasic/Digital first order LPF  Ts=Ts  fcutout=fcc.Fsw/10
  Digital first order LPF2 : pwrsysBasic/Digital first order LPF  Ts=Ts  fcutout=elc.Fsw/10
  Digital first order LPF3 : pwrsysBasic/Digital first order LPF  Ts=Ts  fcutout=btc.Fsw/5
  Digital first order LPF5 : pwrsysBasic/Digital first order LPF  Ts=Ts  fcutout=elc.Pfdroop.UdcComp.Fcutout
  Digital first order LPF6 : pwrsysBasic/Digital first order LPF  Ts=Ts  fcutout=500
  Digital first order LPF7 : pwrsysBasic/Digital first order LPF  Ts=Ts  fcutout=500
  Digital first order LPF8 : pwrsysBasic/Digital first order LPF  Ts=Ts  fcutout=fcc.Pfdroop.UdcComp.Fcutout
  Discrete-Time Integrator : DiscreteIntegrator  IntegratorMethod=Integration: Trapezoidal  ExternalReset=level  InitialConditionSource=external  InitialConditionSetting=State (most efficient)  SampleTime=Ts  LimitOutput=on  UpperSaturationLimit=BT.E_Wh*3600  LowerSaturationLimit=0  ICPrevOutput=DiscIntNeverNeededParam  ICPrevScaledInput=DiscIntNeverNeededParam
  "Droop_controller " : pwrsys-matlab/pwrsysBasic/Droop_controller   Ts=Ts  Outmax=1  Outmin=-1  Refmax=1.5e6/btc.Pn  Refmin=-1.5e6/btc.Pn  Kd=btc.Pfdroop.Kd  Tr=btc.Pfdroop.Tr  flp=btc.Pfdroop.flp  DB=btc.Pfdroop.DB  flp_comp=btc.Pfdroop.UdcComp.Fcutout  Compmax=btc.Pfdroop.UdcComp.udcMax  Compini=1  Compmin=btc.Pfdroop.UdcComp.udcMin
  EL Droop controller : pwrsysBasic/Droop controller  Refmax=0  Refmin=-1  Ts=Ts  Kp=0  Kd=0  Tr=1  flp=1  DB=0
  EL current control : pwrsysVICtrl/Uac_Controller  Ts=Ts  Kg=elc.CurrCont.Kg  Kp=elc.CurrCont.Kp  Ti=elc.CurrCont.Ti  PI_max=elc.CurrCont.PImax  PI_min=elc.CurrCont.PImin
  ELY Current : powerlib/Measurements/Current Measurement  PhasorSimulation=off  OutputType=Complex  PSBequivalent=0
  ELY converter : powerlib/Electrical Sources/Controlled Voltage Source  Initialize=on  Source_Type=DC  Amplitude=fcc.Udc  Phase=0  Frequency=0  Measurements=None
  ELY filter : powerlib/Elements/Series RLC Branch  LConnTagsString=__new0  RConnTagsString=__new0  BranchType=RL  Resistance=elc.filter.R  Inductance=elc.filter.L  SetiL0=on  InitialCurrent=0  Capacitance=1e-6  Setx0=off  InitialVoltage=0  Measurements=None
  ELY output : powerlib/Electrical Sources/Controlled Voltage Source  Initialize=on  Source_Type=DC  Amplitude=fcc.Udc  Phase=0  Frequency=0  Measurements=None
  FC Current : powerlib/Measurements/Current Measurement  PhasorSimulation=off  OutputType=Complex  PSBequivalent=0
  FC Droop controller : pwrsysBasic/Droop controller  Refmax=1  Refmin=0  Ts=Ts  Kp=0  Kd=0  Tr=1  flp=1  DB=0
  FC converter : powerlib/Electrical Sources/Controlled Voltage Source  Initialize=on  Source_Type=DC  Amplitude=fcc.Udc  Phase=0  Frequency=0  Measurements=None
  FC current control : pwrsysVICtrl/Uac_Controller  Ts=Ts  Kg=fcc.CurrCont.Kg  Kp=fcc.CurrCont.Kp  Ti=fcc.CurrCont.Ti  PI_max=fcc.CurrCont.PImax  PI_min=fcc.CurrCont.PImin
  FC filter : powerlib/Elements/Series RLC Branch  LConnTagsString=__new0  RConnTagsString=__new0  BranchType=RL  Resistance=fcc.filter.R  Inductance=fcc.filter.L  SetiL0=on  InitialCurrent=0  Capacitance=1e-6  Setx0=off  InitialVoltage=0  Measurements=None
  FC output : powerlib/Electrical Sources/Controlled Voltage Source  Initialize=on  Source_Type=DC  Amplitude=fcc.Udc  Phase=0  Frequency=0  Measurements=None
  Gain : Gain  Gain=1/ess.Idc
  Gain1 : Gain  Gain=1; %elc.Udc/ess.Udc
  Gain10 : Gain  Gain=1/elc.Udc
  Gain11 : Gain  Gain=1/elc.Udc
  Gain12 : Gain  Gain=btc.Udc/btc.Pn
  Gain13 : Gain  Gain=1/btc.Udc
  Gain14 : Gain  Gain=1/btc.Udc
  Gain15 : Gain  Gain=fcc.Udc/fcc.Pn
  Gain16 : Gain  Gain=elc.Udc/elc.Pn
  Gain17 : Gain  Gain=1/elc.Udc
  Gain18 : Gain  Gain=1/fcc.Udc
  Gain19 : Gain  Gain=3600
  Gain2 : Gain  Gain=1/ess.Idc
  Gain20 : Gain  Gain=-btc.Udc
  Gain21 : Gain  Gain=1/(BT.E_Wh*3600)
  Gain22 : Gain  Gain=BT.UdcSOCfallrate
  Gain3 : Gain  Gain=1; %fcc.Udc/ess.Udc
  Gain4 : Gain  Gain=1/ess.Udc
  Gain5 : Gain  Gain=1/sm.Vn_phase/2^0.5
  Gain6 : Gain  Gain=1; %btc.Udc/ess.Udc
  Gain7 : Gain  Gain=1/fcc.Udc
  Gain8 : Gain  Gain=1/fcc.Udc
  Gain9 : Gain  Gain=1/btc.Udc
  PLL_pu3 : pwrsysBasic/PLL_pu  fn=systemBase.fn  Ts=ess.Ts_control  Kp_pll=90  Ki_pll=1200  Kd_pll=0  PLL_ini=60
  PRef_EL_pu : Sum
  PRef_FC_pu : Sum
  Product : Product  Inputs=3
  Product{1..3,5,7..19} (17 alike) : Product
  Product4 : Product  Inputs=3
  Product6 : Product  Inputs=3
  Rate Limiter : RateLimiter  RisingSlewLimit=fcc.Iref.rise  FallingSlewLimit=fcc.Iref.fall  SampleTimeMode=inherited
  Rate Limiter1 : RateLimiter  RisingSlewLimit=btc.Iref.rise  FallingSlewLimit=btc.Iref.fall  SampleTimeMode=inherited
  Rate Limiter2 : RateLimiter  RisingSlewLimit=elc.Iref.rise  FallingSlewLimit=elc.Iref.fall  SampleTimeMode=inherited
  Relational Operator : RelationalOperator  Operator=>  OutDataTypeStr=boolean
  Relational Operator1 : RelationalOperator  Operator=>  OutDataTypeStr=boolean
  Relational Operator2 : RelationalOperator  Operator=<  OutDataTypeStr=boolean
  Relational Operator3 : RelationalOperator  Operator=<  OutDataTypeStr=boolean
  S-R Flip-Flop : simulink_extras/Flip Flops/S-R Flip-Flop  initial_condition=0
  S-R Flip-Flop1 : simulink_extras/Flip Flops/S-R Flip-Flop  initial_condition=0
  Saturation Dynamic : simulink/Discontinuities/Saturation Dynamic  OutMin=[]  OutMax=[]  OutDataTypeStr=Inherit: Same as second input  OutDataType=fixdt(1, 16)  OutScaling=2^-10  DoSatur=off
  Saturation4 : Saturate  UpperLimit=elc.Pfdroop.UdcComp.udcMax  LowerLimit=elc.Pfdroop.UdcComp.udcMin
  Saturation5 : Saturate  UpperLimit=fcc.Pfdroop.UdcComp.udcMax  LowerLimit=fcc.Pfdroop.UdcComp.udcMin
  Step1 : Step  Time=ess.DCL.deltaTini  SampleTime=Ts
  Step2 : Step  Time=ess.DCL.deltaTini  Before=1  After=0  SampleTime=Ts
  Step3 : Step  Time=ess.DCL.deltaTini  After=-1  SampleTime=Ts
  Sum{,4..6} (4 alike) : Sum  Inputs=|++
  Sum1 : Sum  Inputs=++|
  Sum2 : Sum  Inputs=++|
  Sum3 : Sum  Inputs=+-
  Switch : Switch  Criteria=u2 > Threshold
  Switch1 : Switch  Criteria=u2 > Threshold
  Switch2 : Switch  Threshold=0.5
  Switch3 : Switch  Threshold=0.5
  Terminator : Terminator
  Terminator1 : Terminator
  Terminator2 : Terminator
  Unit Delay1 : UnitDelay  InitialCondition=fcc.Udc  SampleTime=Ts
  Unit Delay2 : UnitDelay  InitialCondition=elc.Udc  SampleTime=Ts
  Unit Delay3 : UnitDelay  InitialCondition=btc.Udc  SampleTime=Ts
  Unit Delay4 : UnitDelay  InitialCondition=btc.Udc  SampleTime=Ts
  Unit Delay5 : UnitDelay  InitialCondition=elc.Udc  SampleTime=Ts
  Unit Delay6 : UnitDelay  InitialCondition=fcc.Udc  SampleTime=Ts
  Unit Delay7 : UnitDelay  InitialCondition=btc.Udc  SampleTime=Ts
  Unit Delay8 : UnitDelay  InitialCondition=0.5  SampleTime=Ts
  Voltage Measurement : powerlib/Measurements/Voltage Measurement  PhasorSimulation=off  OutputType=Complex  PSBequivalent=0
  fromGUI1 : InportShadow  Port=3
  fromGUI2 : InportShadow  Port=3
  fromGUI3 : InportShadow  Port=3
  fromSecCtrl2 : InportShadow  Port=5
  guiPushButtonInterface : Subsystem
  wref : Constant  SampleTime=Ts
  m : Outport
  Idc : Outport  Port=2
  Vdc : Outport  Port=3
  wires:
  [FC_Iref_pu] -> FC current control/1
  [FC_cur_DClink] -> DC-Link Model/1(FC_Idc)
  FC current control/1 -> Product/3, Product8/2  "D"
  [FC_voltage] -> FC output/1
  Bus Selector15/1 -> [ESSPhil_enable]  "<ESSPHIL_enable>"
  Gain/1 -> Product1/1, Bus Creator/2  "DCL_Idc_pu"
  DC-Link Model/2(DCL_Vdc) -> [DCL_Vdc], Vdc/1
  Bus Creator/1 -> m/1
  [DCL_Vdc] -> Gain4/1
  DC-Link Model/1(DCL_Idc) -> [DCL_Idc_pu], Idc/1
  [DCL_Idc_pu] -> Gain/1
  fromGUI/1 -> Bus Selector15/1  "fromGUI"
  Gain4/1 -> Product1/2, Bus Creator/1  "DCL_Vdc_pu"
  Product/1 -> Unit Delay1/1
  [DCL_Vdc] -> Product/2
  fromExtSim/1 -> Bus Selector/1
  Bus Selector1/1 -> Digital first order LPF6/1  "<FC_voltage>"
  Bus Selector1/2 -> Digital first order LPF7/1  "<ELY_voltage>"
  PRef_FC_pu/1 -> FC Droop controller/2  "FC Pref pu"
  FC Droop controller/1 -> Rate Limiter/1
  [FC_current_pu] -> Product3/2, Bus Creator/4  "FC_Idc_pu"
  [ELY_current_pu] -> Product5/2, Bus Creator/8  "ELY_Idc_pu"
  Gain7/1 -> Product3/1, Bus Creator/5  "FC_Vdc_pu"
  Gain10/1 -> Product5/1, Bus Creator/9  "ELY_Vdc_pu"
  [BT_current_pu] -> Product7/2, Bus Creator/12  "BT_Idc_pu"
  Gain13/1 -> Product7/1, Bus Creator/13  "BT_Vdc_pu"
  [ELY_cur_DClink] -> DC-Link Model/2(ELY_Idc)
  [BT_cur_DClink] -> DC-Link Model/3(Batt_Idc)
  Gain8/1 -> Bus Creator/6  "FCC_Vdc_pu"
  Gain11/1 -> Bus Creator/10  "ELC_Vdc_pu"
  Gain14/1 -> Bus Creator/14  "BTC_Vdc_pu"
  Sum5/1 -> [FCC_voltage], FC converter/1
  Constant7/1 -> FC current control/4, FC current control/3
  [FC_voltage] -> Gain7/1
  [FCC_voltage] -> Gain8/1
  [ELY_voltage] -> Gain10/1
  [ELC_voltage] -> Gain11/1
  [BT_voltage] -> Gain13/1
  [BTC_voltage] -> Gain14/1
  [ELY_Iref_pu] -> EL current control/1
  EL current control/1 -> Product9/2, Product4/3  "D"
  [ELY_voltage] -> ELY output/1  "EL_V"
  [ELY_current_pu] -> EL current control/2
  Product4/1 -> Unit Delay2/1
  [DCL_Vdc] -> Product4/2
  Sum4/1 -> ELY converter/1, [ELC_voltage]  "ELC_V"
  Constant3/1 -> EL current control/4, EL current control/3
  [BT_Iref_pu] -> BT current control/1
  BT current control/1 -> Product6/3, Product10/2  "D"
  Product19/1 -> BT output/1
  Product6/1 -> Unit Delay3/1
  [DCL_Vdc] -> Product6/2
  Sum/1 -> [BTC_voltage], BT converter/1
  wref/1 -> Sum3/2
  Sum3/1 -> Product16/2  "delta w"
  Switch1/1 -> Bus Selector1/1
  Bus Creator1/1 -> Switch1/3
  Constant9/1 -> Bus Creator1/1  "FC_voltage"
  Constant10/1 -> Bus Creator1/2  "ELY_voltage"
  Bus Selector15/2 -> [EXTSimEn]  "<ExtSim_enable>"
  Bus Selector/1 -> Switch1/1
  Constant4/1 -> BT current control/4, BT current control/3
  [BT_current_pu] -> BT current control/2  "ib"
  [FC_current_pu] -> FC current control/2
  Product8/1 -> [FC_cur_DClink]
  Product9/1 -> [ELY_cur_DClink]
  Product10/1 -> [BT_cur_DClink]
  [One_After_T] -> EL current control/5
  [One_After_T] -> BT current control/5
  [One_After_T] -> FC current control/5
  Gain15/1 -> Digital first order LPF1/1
  Gain16/1 -> Digital first order LPF2/1
  Gain12/1 -> Digital first order LPF3/1
  Vdc_meas/1 -> DC-Link Model/4(EGSTON_Vdc)
  Product12/1 -> PRef_FC_pu/2
  Gain1/1 -> Product9/1
  Gain3/1 -> Product8/1
  Gain6/1 -> Product10/1
  FC Current/1 -> Gain15/1, Gain3/1
  ELY Current/1 -> Gain16/1, Gain1/1  "EL_I"
  BT Current/1 -> Gain6/1, Gain12/1
  Digital first order LPF6/1 -> [FC_voltage]
  Digital first order LPF7/1 -> [ELY_voltage]
  Digital first order LPF1/1 -> [FC_current_pu]
  Digital first order LPF2/1 -> [ELY_current_pu]
  Digital first order LPF3/1 -> [BT_current_pu]
  Product1/1 -> Bus Creator/3  "DCL_Pdc_pu"
  Product3/1 -> Bus Creator/7  "FC_Pdc_pu"
  Product5/1 -> Bus Creator/11  "EL_Pdc_pu"
  Product7/1 -> Bus Creator/15  "BT_Pdc_pu"
  Bus Selector5/1 -> PRef_FC_pu/1  "<PRef_FC_pu>"
  fromGUI2/1 -> Bus Selector5/1  "fromGUI"
  Bus Selector5/2 -> Product12/1  "<secCtrl_enable>"
  fromSecCtrl/1 -> Bus Selector6/1
  Bus Selector6/1 -> Product12/2  "<Psec_fc>"
  PRef_EL_pu/1 -> EL Droop controller/2  "EL Pref pu"
  EL Droop controller/1 -> Rate Limiter2/1
  Product14/1 -> PRef_EL_pu/2
  Bus Selector7/1 -> PRef_EL_pu/1  "<PRef_ELY_pu>"
  fromGUI3/1 -> Bus Selector7/1  "fromGUI"
  Bus Selector7/2 -> Product14/1  "<secCtrl_enable>"
  fromSecCtrl2/1 -> Bus Selector8/1
  Bus Selector8/1 -> Product14/2  "<Psec_ely>"
  fromESS/1 -> Bus Selector2/1
  Bus Selector4/1 -> Product11/1  "<PRef_Batt_pu>"
  fromGUI1/1 -> Bus Selector4/1  "fromGUI"
  Product11/1 -> "Droop_controller "/5
  Bus Selector2/1 -> DC-Link Model/5(ESSsim_Vdc)  "<Vdc_pu>"
  Step1/1 -> [One_After_T]
  Step2/1 -> [Zero_After_T]
  Step3/1 -> [MinusOne_After_T]
  Unit Delay3/1 -> Sum/1
  [Zero_After_T] -> Product2/2
  Constant1/1 -> Product2/1
  Product2/1 -> Sum/2
  [Zero_After_T] -> Product13/2
  Constant11/1 -> Product13/1
  Product13/1 -> Sum4/2
  Unit Delay2/1 -> Sum4/1  "EL_V_controller"
  [Zero_After_T] -> Product15/2
  Constant6/1 -> Product15/1
  Product15/1 -> Sum5/2
  Unit Delay1/1 -> Sum5/1
  [Zero_After_T] -> EL current control/6
  Constant12/1 -> EL current control/7
  [Zero_After_T] -> BT current control/6
  Constant18/1 -> BT current control/7
  [Zero_After_T] -> FC current control/6
  Constant19/1 -> FC current control/7
  [One_After_T] -> Product4/1
  [One_After_T] -> Product6/1
  [One_After_T] -> Product/1
  Gain2/1 -> Bus Creator/16  "GC_Idc_pu"
  [DCL_Idc_pu] -> Gain2/1
  Vabc/1 -> Gain5/1
  PLL_pu3/1 -> Terminator1/1
  Gain5/1 -> PLL_pu3/1
  PLL_pu3/2 -> [w_pu]
  [w_pu] -> Sum3/1
  [One_After_T] -> Product11/2
  [BTC_voltage] -> Unit Delay4/1
  Unit Delay4/1 -> Gain9/1
  Constant2/1 -> EL Droop controller/1
  Digital first order LPF5/1 -> Saturation4/1
  [ELC_voltage] -> Unit Delay5/1
  Gain17/1 -> Digital first order LPF5/1
  Unit Delay5/1 -> Gain17/1
  Saturation4/1 -> EL Droop controller/3
  Product16/1 -> "Droop_controller "/1
  [One_After_T] -> Product16/1
  Constant5/1 -> FC Droop controller/1
  Digital first order LPF8/1 -> Saturation5/1
  [FCC_voltage] -> Unit Delay6/1
  Gain18/1 -> Digital first order LPF8/1
  Unit Delay6/1 -> Gain18/1
  Saturation5/1 -> FC Droop controller/3
  Rate Limiter/1 -> [FC_Iref_pu]
  Rate Limiter2/1 -> [ELY_Iref_pu]
  Rate Limiter1/1 -> [BT_Iref_pu]
  Voltage Measurement/1 -> Unit Delay7/1
  Unit Delay7/1 -> [BT_voltage]
  Constant13/1 -> Gain19/1
  Gain19/1 -> Discrete-Time Integrator/3
  Constant14/1 -> Switch/3
  Constant/1 -> Switch/1
  BT Current1/1 -> [BAT_Iint]
  [BAT_Iint] -> Gain20/1
  Gain20/1 -> Discrete-Time Integrator/1
  Discrete-Time Integrator/1 -> Gain21/1
  Gain21/1 -> Unit Delay8/1, [BAT_SOC]
  [BAT_SOC] -> Bus Creator/17  "BAT_SOC"
  [SOC_enable] -> Switch/2
  guiPushButtonInterface/1(Out1) -> Sum1/1
  Switch/1 -> Sum1/2
  Sum1/1 -> Discrete-Time Integrator/2
  [ESSPhil_enable] -> DC-Link Model/6(EGSTON_enable)
  [EXTSimEn] -> Switch1/2
  Bus Selector15/3 -> [SOC_enable]  "<SOC_enable>"
  Bus Selector15/4 -> [resetSOC]  "<resetSOC>"
  [resetSOC] -> guiPushButtonInterface/1(In1)
  Relational Operator/1 -> S-R Flip-Flop/1
  Constant16/1 -> Relational Operator1/1
  Relational Operator1/1 -> S-R Flip-Flop/2
  S-R Flip-Flop/2 -> Data Type Conversion6/1
  Data Type Conversion6/1 -> [underSOCmax]
  S-R Flip-Flop/1 -> Terminator/1
  Relational Operator2/1 -> S-R Flip-Flop1/1
  Relational Operator3/1 -> S-R Flip-Flop1/2
  S-R Flip-Flop1/2 -> Data Type Conversion1/1
  Data Type Conversion1/1 -> [overSOCmin]
  S-R Flip-Flop1/1 -> Terminator2/1
  "Droop_controller "/1 -> Saturation Dynamic/2  "ibref"
  Saturation Dynamic/1 -> Rate Limiter1/1
  Constant21/1 -> Product17/1
  [overSOCmin] -> Product17/2
  Product17/1 -> Saturation Dynamic/1
  Constant22/1 -> Product18/1
  [underSOCmax] -> Product18/2
  Product18/1 -> Saturation Dynamic/3
  [BAT_SOC] -> Relational Operator3/2, Relational Operator2/1, Relational Operator1/2, Relational Operator/1
  Constant15/1 -> Relational Operator/2
  Constant17/1 -> Relational Operator2/2
  Constant20/1 -> Relational Operator3/1
  Constant23/1 -> Sum2/2
  Sum2/1 -> Gain22/1
  Unit Delay8/1 -> Sum2/1
  Constant8/1 -> Product19/1
  Sum6/1 -> Product19/2
  Gain22/1 -> Sum6/1
  Constant24/1 -> Sum6/2
  [FCRNCase2] -> Switch2/2
  Constant25/1 -> Switch2/3
  Constant26/1 -> Switch2/1
  Switch2/1 -> Switch3/3
  [FCRNCase3] -> Switch3/2
  Constant27/1 -> Switch3/1
  Constant30/1 -> "Droop_controller "/3
  Constant31/1 -> "Droop_controller "/4
  Switch3/1 -> [FCRNKp]
  [FCRNKp] -> "Droop_controller "/2
  Gain9/1 -> "Droop_controller "/6
  Bus Selector15/5 -> [FCRNCase2]  "<FCRN_Case2>"
  Bus Selector15/6 -> [FCRNCase3]  "<FCRN_Case3>"
  connections:
  FC output/RConn1 -- FC filter/LConn1
  FC converter/RConn1 -- FC Current/RConn1
  FC filter/RConn1 -- FC Current/LConn1
  FC output/LConn1 -- FC converter/LConn1
  ELY converter/RConn1 -- ELY Current/RConn1
  ELY output/RConn1 -- ELY filter/LConn1
  ELY output/LConn1 -- ELY converter/LConn1
  ELY filter/RConn1 -- ELY Current/LConn1
  BT converter/RConn1 -- BT Current/RConn1
  BT R2/RConn1 -- Voltage Measurement/LConn1 -- BT C/RConn1 -- BT filter/LConn1
  BT filter/RConn1 -- BT Current/LConn1
  BT output/LConn1 -- BT converter/LConn1 -- Voltage Measurement/LConn2
  BT R1/RConn1 -- BT C/LConn1 -- BT R2/LConn1
  BT Current1/RConn1 -- BT R1/LConn1
  BT Current1/LConn1 -- BT output/RConn1
